simulink model "Exercise_2"  (R2024b)
settings: Solver=ode4  StartTime=0.0  StopTime=0.1  FixedStep=0.1  RelTol=1e-3
settings Model: Creator=Roshan Sharma  LastModifiedBy=Torstein
settings SolverCC: AlgebraicLoopSolver=TrustRegion
settings DataIOCC: ReturnWorkspaceOutputs=off
settings DebuggingCC: UnconnectedInputMsg=warning  UnconnectedOutputMsg=warning  UnconnectedLineMsg=warning  ArithmeticOperatorsInVariantConditions=warning
settings ModelReferenceCC: EnableRefExpFcnMdlSchedulingChecks=on
settings SFSimCC: SimUseLocalCustomCode=off  CustomCodeUndefinedFunction=UseInterfaceOnly
settings RTWCC: RTWUseLocalCustomCode=off  GPUComputeCapability=3.5
settings CodeAppCC: StateflowObjectComments=on

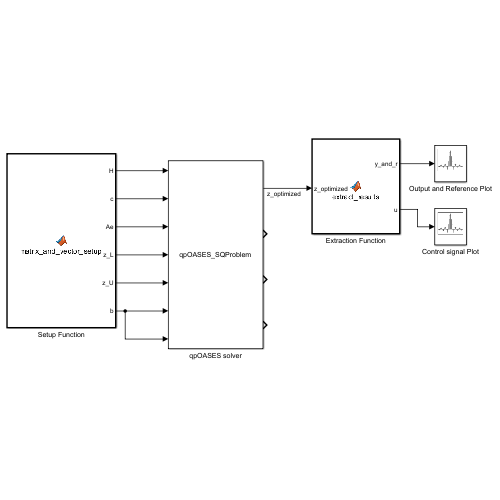
[thumbnail: Simulink's stored preview of the top-level diagram]
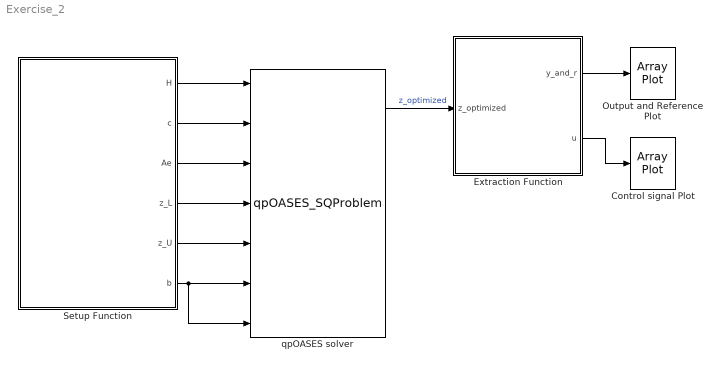
== system Exercise_2 ==
  Control signal Plot : ArrayPlot  WindowPosition=[769.000000,49.000000,766.000000,880.000000,]  ScopeFrameLocation=window  SampleIncrement=0.08333  PlotType=Line  AxesScaling=Manual  XLabel=Time [12/10 s]  YLabel=control input [u]  YLimits=[-14.669708007399578 17.866391992600423]  ShowLegend=on  ChannelNames=['Force applied on the cart']  DefaultConfigurationName=dsp.scopes.ArrayPlotBlockSpecification
  Extraction Function : MATLAB Function  TreatAsAtomicUnit=on
  Output and Reference Plot : ArrayPlot  WindowPosition=[1.000000,49.000000,766.000000,880.000000,]  ScopeFrameLocation=window  PlotType=Line  AxesScaling=Manual  Title=LQ optimal control of inverted pendulum  XLabel=Time steps [k]  YLabel=outputs and setpoints [y, r]  YLimits=[-0.5 3.5]  ShowLegend=on  ChannelNames=['y1: pendulum angle','y2: cart position','r1: pendulum angle set point','r2: cart position set point']  DefaultConfigurationName=dsp.scopes.ArrayPlotBlockSpecification
  Setup Function : MATLAB Function  TreatAsAtomicUnit=on
  qpOASES solver : S-Function  FunctionName=qpOASES_SQProblem  SFunctionDeploymentMode=off  EnableBusSupport=off
  wires:
  Setup Function/1(H) -> qpOASES solver/1
  Setup Function/2(c) -> qpOASES solver/2
  Setup Function/3(Ae) -> qpOASES solver/3
  Setup Function/4(z_L) -> qpOASES solver/4
  Setup Function/5(z_U) -> qpOASES solver/5
  Setup Function/6(b) -> qpOASES solver/7, qpOASES solver/6
  qpOASES solver/1 -> Extraction Function/1(z_optimized)  "z_optimized"
  Extraction Function/1(y_and_r) -> Output and Reference Plot/1
  Extraction Function/2(u) -> Control signal Plot/1

== matlab function Exercise_2/Extraction Function ==
  data: y_and_r output; u output; z_optimized input
function [y_and_r, u] = extract_results(z_optimized)

% Size numbers
N = 120;
nx = 4;
nu = 1;
ny = 2;

% Extract results
ua = z_optimized(1 + N * 0 : N * nu, 1);                                %control inputs
xa = z_optimized(1 + N * nu : N * (nu + nx), :);                        %states
ea = z_optimized(1 + N * (nu + nx) : N * (nu + nx + ny), :);            %error in tracking
ya = z_optimized(1 + N * (nu + nx + ny) : N * (nu + nx + ny + ny), :);  %outputs

y = reshape(ya, ny, N)';

ref_shift = 3;
r = [zeros(N, 1), [zeros(N / 2, 1); ref_shift * ones(N / 2, 1)]];

y_and_r = [y, r(:, 1), r(:, 2)];
u = reshape(ua, nu, N)';

== matlab function Exercise_2/Setup Function ==
  data: H output; c output; Ae output; z_L output; z_U output; b output
function [H, c, Ae, z_L, z_U, b]  = matrix_and_vector_setup
% f = 0.5 z^T H z + c^T z
% z = [x, u, e, y]^T

% Problem matrixes
A = [1.0745, 0.1025, 0, 0;
    1.5079, 1.0745, 0, 0;
    -0.0248, -0.0008, 1, 0.1;
    -0.5026, -0.0248, 0, 1];
B = [-0.0025, -0.0512, 0.0025, 0.0504]';
C = [1, 0, 0, 0;
    0, 0, 1, 0];

N = int32(12 / 0.1); % Number of time points
nx = 4; % Number of states
ny = 2; % Number of outputs
nu = 1; % Number of inputs
nz = N * (nx + nu + 2 * ny); % Total number of model points

x_init = [0, 0, 0, 0]'; % Initial state values

ref_shift = 3;
r = [zeros(1, N); zeros(1, N / 2) ref_shift * ones(1, N / 2)]; % Reference setpoints

Q = diag([1 1]); % Error weight tuning matrix
P = 1e-3; % Input weight tuning matrix

% Hessian matrix
H_1 = kron(eye(N), P);
H_2 = zeros(N * nx, N * nx);
H_3 = kron(eye(N), Q);
H_4 = zeros(N * ny, N * ny);
H_mat = blkdiag(H_1, H_2, H_3, H_4);
H = H_mat(:);

% Single term vector
c = zeros(nz, 1);

% Constraints
A_1u = kron(eye(N), -B);
A_1x = eye(N * nx) - kron(diag(ones(N - abs(-1), 1), -1), A);
A_1e = zeros(N * nx, N * ny);
A_1y = zeros(N * nx, N * ny);
A_2u = zeros(N * ny, N * nu);
A_2x = kron(eye(N), -C);
A_2e = zeros(N * ny, N * ny);
A_2y = eye(N * ny);
A_3u = zeros(N * ny, N * nu);
A_3x = zeros(N * ny, N * nx);
A_3e = eye(N * ny);
A_3y = eye(N * ny);
Ae_mat = [A_1u A_1x A_1e A_1y;
    A_2u A_2x A_2e A_2y;
    A_3u A_3x A_3e A_3y];
Ae = Ae_mat(:);

b_1 = [A * x_init; zeros((N - 1) * nx, 1)];
b_2 = zeros(N * ny, 1);
b_3 = reshape(r, N * ny, 1);
b = [b_1; b_2; b_3];

% Bounds
z_L = - Inf * ones(nz, 1);
z_U = Inf * ones(nz, 1);

end
